simulink model "practica_5_simulink"  (R2026a)
settings: Solver=VariableStepAuto  StopTime=0.003
settings Model: Creator=dante  LastModifiedBy=dante

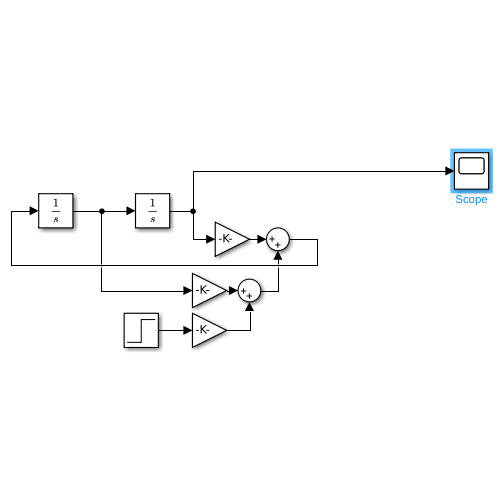
[thumbnail: Simulink's stored preview of the top-level diagram]
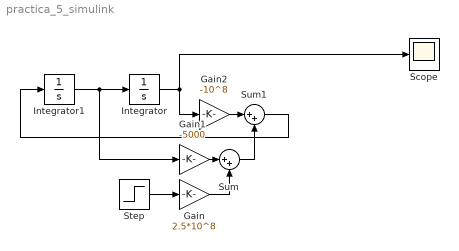
== system practica_5_simulink ==
  Gain : Gain  Gain=2.5*10^8
  Gain1 : Gain  Gain=-5000
  Gain2 : Gain  Gain=-10^8
  Integrator : Integrator  InitialCondition=1
  Integrator1 : Integrator
  Scope : Scope
      settings: ActiveDisplayYMinimum=0.72947062009519814  ActiveDisplayYMaximum=3.4347644191432174
  Step : Step  Time=0  SampleTime=0
  Sum : Sum  Inputs=|++
  Sum1 : Sum  Inputs=|++
  wires:
  Step/1 -> Gain/1
  Integrator1/1 -> Gain1/1, Integrator/1
  Gain/1 -> Sum/2
  Gain1/1 -> Sum/1
  Sum/1 -> Sum1/2
  Gain2/1 -> Sum1/1
  Integrator/1 -> Gain2/1, Scope/1
  Sum1/1 -> Integrator1/1
